simulink library "SimplusGT_2020a"  (R2020a)
settings: Solver=ode45  StartTime=0.0  StopTime=10.0  RelTol=1e-3
undefined symbols (not defined in the file): ang_r, Cf, DiscIntNeverNeededParam, initial, Lc, Lf, m, OtherInputs, P_dc, Sbase, t0, Tm_pu, Ts, V, Vbase, w_droop, w_i, w_pll, w_tau, w_v, Wbase, wc, wfil, x0, Ybase, Zbase
libraries: powerlib x217, $bdroot x1, SimplexPS_2015a x1
(part 3 of 5)

== system SimplusGT_2020a/P-w droop ==
  note: p-w droop controller
      |
      | Author(s): Yitong Li
      |
      | Notes:
      |
      | The power reference should be in source convention.
  pq : Inport
  Constant : Constant  Value=w0
  Constant2 : Constant  Value=theta0
  Constant4 : Constant  Value=2*pi
  Constant6 : Constant  Value=p0
  Demux : Demux  Outputs=2
  Discrete-Time Integrator : DiscreteIntegrator  SampleTime=Ts  ICPrevOutput=DiscIntNeverNeededParam  ICPrevScaledInput=DiscIntNeverNeededParam
  Filter p : DiscreteTransferFcn  Numerator=w_tau*Ts  Denominator=[1 ((w_tau*Ts)-1)]  SampleTime=Ts
  Gain : Gain  Gain=1/Sbase
  Gain2 : Gain  Gain=m
  Gain3 : Gain  Gain=Wbase
  Math Function1 : Math  Operator=mod  SignedPower=on  SaturateOnIntegerOverflow=on
  Sum : Sum
  Sum1 : Sum
  Sum2 : Sum  Inputs=+-
  w : Outport
  theta : Outport  Port=2
  wires:
  Gain3/1 -> Discrete-Time Integrator/1, w/1, [w]
  Sum/1 -> Gain3/1
  Sum2/1 -> Gain2/1
  Constant6/1 -> Sum2/1
  pq/1 -> Demux/1
  Constant4/1 -> Math Function1/2
  Constant/1 -> Sum/2
  Filter p/1 -> Sum2/2
  Discrete-Time Integrator/1 -> Sum1/1
  Gain2/1 -> Sum/1
  Math Function1/1 -> theta/1, [theta]
  Constant2/1 -> [theta0], Sum1/2
  Sum1/1 -> Math Function1/1
  Demux/1 -> Gain/1  "p"
  Gain/1 -> Filter p/1

== system SimplusGT_2020a/PLL (vDQ -> vq) ==
  note: Gpll
  note: Measurement
  note: Phase lock loop (PLL)
      |
      | Author(s): Yitong Li
      |
      | Notes:
      |
      | vq is fed into the PI controller of the PLL.
      |
      | This PLL assumes the input voltage is in DQ frame, which is the common electrical frame. It is not a practical PLL which uses vabc as the input. But this PLL is useful in research.
  vDQ : Inport
  wDQ : Inport  Port=2
  Constant1 : Constant
  Constant2 : Constant  Value=theta0
  Constant3 : Constant
  Constant4 : Constant  Value=2*pi
  Constant6 : Constant  Value=0
  Demux1 : Demux  Outputs=2
  Discrete PI1 : Subsystem  AncestorBlock=SimplusGT/Discrete PI  mask{Kp=w_pll, Ki=w_pll*w_pll/4, xmax=inf, xmin=-inf, Ts=Ts}
      mask prompts: Kp "Proportional Gain"; Ki "Integral Gain"; xmax "Upper Limit"; xmin "Lower Limit"; Ts "Sampling Time"
  Discrete-Time Integrator : DiscreteIntegrator  SampleTime=Ts  ICPrevOutput=DiscIntNeverNeededParam  ICPrevScaledInput=DiscIntNeverNeededParam
  Filter p : DiscreteTransferFcn  Numerator=w_tau*Ts  Denominator=[1 ((w_tau*Ts)-1)]  SampleTime=Ts
  Gain1 : Gain  Gain=Wbase
  Gain2 : Gain  Gain=1/Vbase
  Gain4 : Gain  Gain=1/Wbase
  Gain5 : Gain  Gain=1/pi
  Math Function1 : Math  Operator=mod  SignedPower=on  SaturateOnIntegerOverflow=on
  Mux : Mux  Inputs=2
  Scope : Scope  NumInputPorts=4
  Sum : Sum
  Sum1 : Sum
  Sum2 : Sum  Inputs=+-
  "x1y1 -> x2y2" : Subsystem  AncestorBlock=SimplusGT/x1y1 -> x2y2
  wdq : Outport
  theta : Outport  Port=2
  vdq : Outport  Port=3
  wires:
  [theta0] -> Mux/1  "theta0"
  Constant2/1 -> [theta0], Sum1/2
  Math Function1/1 -> "x1y1 -> x2y2"/2(theta), theta/1, [theta]
  Sum1/1 -> Math Function1/1
  Demux1/2 -> [vq], Gain2/1
  vDQ/1 -> "x1y1 -> x2y2"/1(x1y1)
  Discrete-Time Integrator/1 -> Sum1/1
  Gain2/1 -> Filter p/1
  [vd] -> Scope/1  "vd"
  Mux/1 -> Gain5/1
  Discrete PI1/1(Out) -> Sum/1
  "x1y1 -> x2y2"/1(x2y2) -> vdq/1, Demux1/1
  [w] -> Gain4/1  "w"
  Constant4/1 -> Math Function1/2
  [theta] -> Mux/2  "theta"
  Demux1/1 -> [vd]
  Gain5/1 -> Scope/4
  Constant1/1 -> Discrete PI1/1(enable)
  Gain4/1 -> Scope/3
  Gain1/1 -> Sum/2
  Constant3/1 -> Gain1/1
  [vq] -> Scope/2  "vq"
  Filter p/1 -> Discrete PI1/2(reference)
  Constant6/1 -> Discrete PI1/4(actual), Discrete PI1/3(initial)
  Sum/1 -> Sum2/1
  Sum2/1 -> [w], wdq/1, Discrete-Time Integrator/1
  wDQ/1 -> Sum2/2

== system SimplusGT_2020a/PLL (vabc -> theta) ==
  note: Measurement
  note: Gpll
  note: Phase lock loop (PLL)
      |
      | Author(s): Yitong Li
      |
      | Notes:
      |
      | theta of voltage is fed into the PI controller of the PLL.
  vabc : Inport
  Constant1 : Constant
  Constant2 : Constant  Value=2*pi
  Constant3 : Constant  Value=0
  Constant4 : Constant
  Constant5 : Constant  Value=theta0
  Demux : Demux  Outputs=2
  Discrete PI : Subsystem  AncestorBlock=SimplusGT/Discrete PI  mask{Kp=w_pll, Ki=w_pll*w_pll/4, xmax=inf, xmin=-inf, Ts=Ts}
      mask prompts: Kp "Proportional Gain"; Ki "Integral Gain"; xmax "Upper Limit"; xmin "Lower Limit"; Ts "Sampling Time"
  Discrete-Time Integrator : DiscreteIntegrator  SampleTime=Ts  ICPrevOutput=DiscIntNeverNeededParam  ICPrevScaledInput=DiscIntNeverNeededParam
  Filter p : DiscreteTransferFcn  Numerator=w_tau*Ts  Denominator=[1 ((w_tau*Ts)-1)]  SampleTime=Ts
  Gain1 : Gain  Gain=Wbase
  Gain4 : Gain  Gain=1/Wbase
  Gain5 : Gain  Gain=1/pi
  Math Function1 : Math  Operator=mod  SignedPower=on  SaturateOnIntegerOverflow=on
  Mux : Mux  Inputs=2
  Scope : Scope  NumInputPorts=4
  Selector : Selector  InputPortWidth=2  IndexOptions=Index vector (dialog)  Indices=[2 1]  OutputSizes=1
  Sum : Sum
  Sum1 : Sum
  Trigonometric Function : Trigonometry  Operator=atan2
  "abc -> dq (Power-Invariant)" : Subsystem  AncestorBlock=|
      | SimplusGT/abc -> dq
      | (Power-Invariant)
  w : Outport
  theta : Outport  Port=2
  vdq : Outport  Port=3
  wires:
  Constant2/1 -> Math Function1/2
  Constant1/1 -> Discrete PI/1(enable)
  Constant3/1 -> Discrete PI/3(initial), Discrete PI/4(actual)
  Trigonometric Function/1 -> Filter p/1
  Demux/1 -> [vq], Trigonometric Function/1
  Demux/2 -> [vd], Trigonometric Function/2
  Selector/1 -> Demux/1
  Math Function1/1 -> "abc -> dq (Power-Invariant)"/2(theta), [theta], theta/1
  "abc -> dq (Power-Invariant)"/1(dq) -> vdq/1, Selector/1
  vabc/1 -> "abc -> dq (Power-Invariant)"/1(abc)
  Discrete PI/1(Out) -> Sum/1
  Constant4/1 -> Gain1/1
  Sum/1 -> [w], w/1, Discrete-Time Integrator/1
  Filter p/1 -> Discrete PI/2(reference)
  [vq] -> Scope/2  "vq"
  Mux/1 -> Gain5/1
  [vd] -> Scope/1  "vd"
  [theta] -> Mux/2  "theta"
  Gain5/1 -> Scope/4
  Gain4/1 -> Scope/3
  [w] -> Gain4/1  "w"
  [theta0] -> Mux/1  "theta0"
  Gain1/1 -> Sum/2
  Discrete-Time Integrator/1 -> Sum1/1
  Sum1/1 -> Math Function1/1
  Constant5/1 -> [theta0], Sum1/2

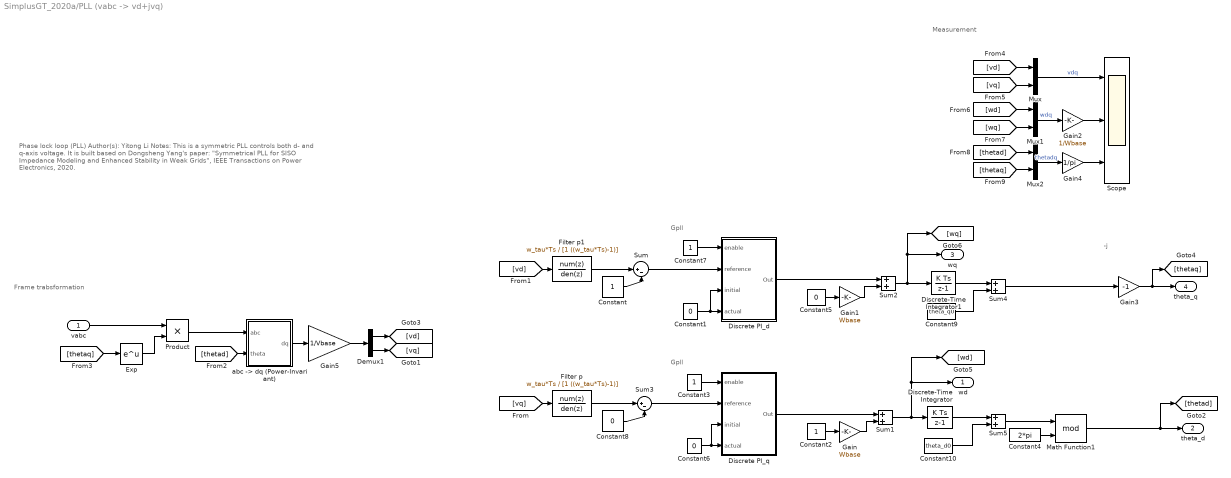
== system SimplusGT_2020a/PLL (vabc -> vd+jvq) ==
  note: Measurement
  note: Frame trabsformation
  note: -j
  note: Gpll
  note: Gpll
  note: Phase lock loop (PLL)
      |
      | Author(s): Yitong Li
      |
      | Notes:
      |
      | This is a symmetric PLL controls both d- and q-axis voltage.
      |
      | It is built based on Dongsheng Yang's paper: "Symmetrical PLL for SISO Impedance Modeling and Enhanced Stability in Weak Grids", IEEE Transactions on Power Electronics, 2020.
  vabc : Inport
  Constant{,2..3,7} (4 alike) : Constant
  Constant{1,5..6,8} (4 alike) : Constant  Value=0
  Constant10 : Constant  Value=theta_d0
  Constant4 : Constant  Value=2*pi
  Constant9 : Constant  Value=theta_q0
  Demux1 : Demux  Outputs=2
  Discrete PI_d : Subsystem  AncestorBlock=SimplusGT/Discrete PI  mask{Kp=w_pll, Ki=w_pll*w_pll/4, xmax=inf, xmin=-inf, Ts=Ts}
      mask prompts: Kp "Proportional Gain"; Ki "Integral Gain"; xmax "Upper Limit"; xmin "Lower Limit"; Ts "Sampling Time"
  Discrete PI_q : Subsystem  AncestorBlock=SimplusGT/Discrete PI  mask{Kp=w_pll, Ki=w_pll*w_pll/4, xmax=inf, xmin=-inf, Ts=Ts}
      mask prompts: Kp "Proportional Gain"; Ki "Integral Gain"; xmax "Upper Limit"; xmin "Lower Limit"; Ts "Sampling Time"
  Discrete-Time Integrator : DiscreteIntegrator  SampleTime=Ts  ICPrevOutput=DiscIntNeverNeededParam  ICPrevScaledInput=DiscIntNeverNeededParam
  Discrete-Time Integrator1 : DiscreteIntegrator  SampleTime=Ts  ICPrevOutput=DiscIntNeverNeededParam  ICPrevScaledInput=DiscIntNeverNeededParam
  Exp : Math  SignedPower=on  SaturateOnIntegerOverflow=on
  Filter p : DiscreteTransferFcn  Numerator=w_tau*Ts  Denominator=[1 ((w_tau*Ts)-1)]  SampleTime=Ts
  Filter p1 : DiscreteTransferFcn  Numerator=w_tau*Ts  Denominator=[1 ((w_tau*Ts)-1)]  SampleTime=Ts
  Gain : Gain  Gain=Wbase
  Gain1 : Gain  Gain=Wbase
  Gain2 : Gain  Gain=1/Wbase
  Gain3 : Gain  Gain=-1
  Gain4 : Gain  Gain=1/pi
  Gain5 : Gain  Gain=1/Vbase
  Math Function1 : Math  Operator=mod  SignedPower=on  SaturateOnIntegerOverflow=on
  Mux : Mux  Inputs=2
  Mux1 : Mux  Inputs=2
  Mux2 : Mux  Inputs=2
  Product : Product
  Scope : Scope  NumInputPorts=3
  Sum : Sum  Inputs=|+-
  Sum{1..2,4..5} (4 alike) : Sum
  Sum3 : Sum  Inputs=|+-
  "abc -> dq (Power-Invariant)" : Subsystem  AncestorBlock=|
      | SimplusGT/abc -> dq
      | (Power-Invariant)
  wd : Outport
  theta_d : Outport  Port=2
  wq : Outport  Port=3
  theta_q : Outport  Port=4
  wires:
  Constant4/1 -> Math Function1/2
  Constant6/1 -> Discrete PI_q/3(initial), Discrete PI_q/4(actual)
  Demux1/2 -> [vq]
  Constant3/1 -> Discrete PI_q/1(enable)
  Math Function1/1 -> theta_d/1, [thetad]
  "abc -> dq (Power-Invariant)"/1(dq) -> Gain5/1
  Gain5/1 -> Demux1/1
  Demux1/1 -> [vd]
  Constant/1 -> Sum/2
  Sum/1 -> Discrete PI_d/2(reference)
  Constant7/1 -> Discrete PI_d/1(enable)
  Constant1/1 -> Discrete PI_d/4(actual), Discrete PI_d/3(initial)
  [thetad] -> "abc -> dq (Power-Invariant)"/2(theta)
  vabc/1 -> Product/1
  Product/1 -> "abc -> dq (Power-Invariant)"/1(abc)
  Exp/1 -> Product/2
  Gain3/1 -> theta_q/1, [thetaq]
  [vq] -> Filter p/1
  [vd] -> Filter p1/1
  Filter p1/1 -> Sum/1
  [thetaq] -> Exp/1
  Sum1/1 -> [wd], wd/1, Discrete-Time Integrator/1
  Discrete PI_q/1(Out) -> Sum1/1
  Sum2/1 -> Discrete-Time Integrator1/1, wq/1, [wq]
  Discrete PI_d/1(Out) -> Sum2/1
  Constant2/1 -> Gain/1
  Constant5/1 -> Gain1/1
  Filter p/1 -> Sum3/1
  Constant8/1 -> Sum3/2
  Sum3/1 -> Discrete PI_q/2(reference)
  Discrete-Time Integrator1/1 -> Sum4/1
  Sum4/1 -> Gain3/1
  Constant9/1 -> Sum4/2
  Gain/1 -> Sum1/2
  Gain1/1 -> Sum2/2
  Discrete-Time Integrator/1 -> Sum5/1
  Sum5/1 -> Math Function1/1
  Constant10/1 -> Sum5/2
  [vd] -> Mux/1
  [vq] -> Mux/2
  [wd] -> Mux1/1
  [wq] -> Mux1/2
  [thetad] -> Mux2/1
  [thetaq] -> Mux2/2
  Mux/1 -> Scope/1  "vdq"
  Mux1/1 -> Gain2/1  "wdq"
  Mux2/1 -> Gain4/1  "thetadq"
  Gain2/1 -> Scope/2
  Gain4/1 -> Scope/3

== system SimplusGT_2020a/PLL (vabc -> vq) ==
  note: Measurement
  note: Gpll
  note: Phase lock loop (PLL)
      |
      | Author(s): Yitong Li
      |
      | Notes:
      |
      | vq is fed into the PI controller of the PLL.
  vabc : Inport
  Constant1 : Constant
  Constant2 : Constant  Value=theta0
  Constant3 : Constant
  Constant4 : Constant  Value=2*pi
  Constant6 : Constant  Value=0
  Demux1 : Demux  Outputs=2
  Discrete PI : Subsystem  AncestorBlock=SimplusGT/Discrete PI  mask{Kp=w_pll, Ki=w_pll*w_pll/4, xmax=inf, xmin=-inf, Ts=Ts}
      mask prompts: Kp "Proportional Gain"; Ki "Integral Gain"; xmax "Upper Limit"; xmin "Lower Limit"; Ts "Sampling Time"
  Discrete-Time Integrator : DiscreteIntegrator  SampleTime=Ts  ICPrevOutput=DiscIntNeverNeededParam  ICPrevScaledInput=DiscIntNeverNeededParam
  Filter p : DiscreteTransferFcn  Numerator=w_tau*Ts  Denominator=[1 ((w_tau*Ts)-1)]  SampleTime=Ts
  Gain1 : Gain  Gain=Wbase
  Gain2 : Gain  Gain=1/Vbase
  Gain4 : Gain  Gain=1/Wbase
  Gain5 : Gain  Gain=1/pi
  Math Function1 : Math  Operator=mod  SignedPower=on  SaturateOnIntegerOverflow=on
  Mux : Mux  Inputs=2
  Scope : Scope  NumInputPorts=4
  Sum : Sum
  Sum1 : Sum
  "abc -> dq (Power-Invariant)" : Subsystem  AncestorBlock=|
      | SimplusGT/abc -> dq
      | (Power-Invariant)
  w : Outport
  theta : Outport  Port=2
  vdq : Outport  Port=3
  wires:
  vabc/1 -> "abc -> dq (Power-Invariant)"/1(abc)
  "abc -> dq (Power-Invariant)"/1(dq) -> vdq/1, Demux1/1
  Constant4/1 -> Math Function1/2
  Gain2/1 -> Filter p/1
  Demux1/2 -> [vq], Gain2/1
  Constant6/1 -> Discrete PI/4(actual), Discrete PI/3(initial)
  Constant1/1 -> Discrete PI/1(enable)
  Discrete PI/1(Out) -> Sum/1
  Sum/1 -> [w], w/1, Discrete-Time Integrator/1
  Gain1/1 -> Sum/2
  Discrete-Time Integrator/1 -> Sum1/1
  Sum1/1 -> Math Function1/1
  Constant2/1 -> [theta0], Sum1/2
  Filter p/1 -> Discrete PI/2(reference)
  [vq] -> Scope/2  "vq"
  Mux/1 -> Gain5/1
  Gain4/1 -> Scope/3
  [w] -> Gain4/1  "w"
  [theta0] -> Mux/1  "theta0"
  [vd] -> Scope/1  "vd"
  Gain5/1 -> Scope/4
  [theta] -> Mux/2  "theta"
  Demux1/1 -> [vd]
  Constant3/1 -> Gain1/1
  Math Function1/1 -> "abc -> dq (Power-Invariant)"/2(theta), [theta], theta/1

== system SimplusGT_2020a/PQ Calculation (dq-Frame) ==
  note: Power calculation.
      |
      | Author(s): Yitong Li
      |
      | Notes:
      |
      | The calculation is done in dq frame.
  vdq : Inport
  idq : Inport  Port=2
  Mux : Mux  Inputs=2
  Mux1 : Mux  Inputs=2
  P = vd*id+vq*iq : Fcn  Expr=u[1]*u[3]+u[2]*u[4]
  Q = -vd*iq+vq*id : Fcn  Expr=-u[1]*u[4]+u[2]*u[3]
  pq : Outport
  wires:
  Q = -vd*iq+vq*id/1 -> Mux/2
  Mux1/1 -> Q = -vd*iq+vq*id/1, P = vd*id+vq*iq/1
  idq/1 -> Mux1/2
  vdq/1 -> Mux1/1
  P = vd*id+vq*iq/1 -> Mux/1
  Mux/1 -> pq/1

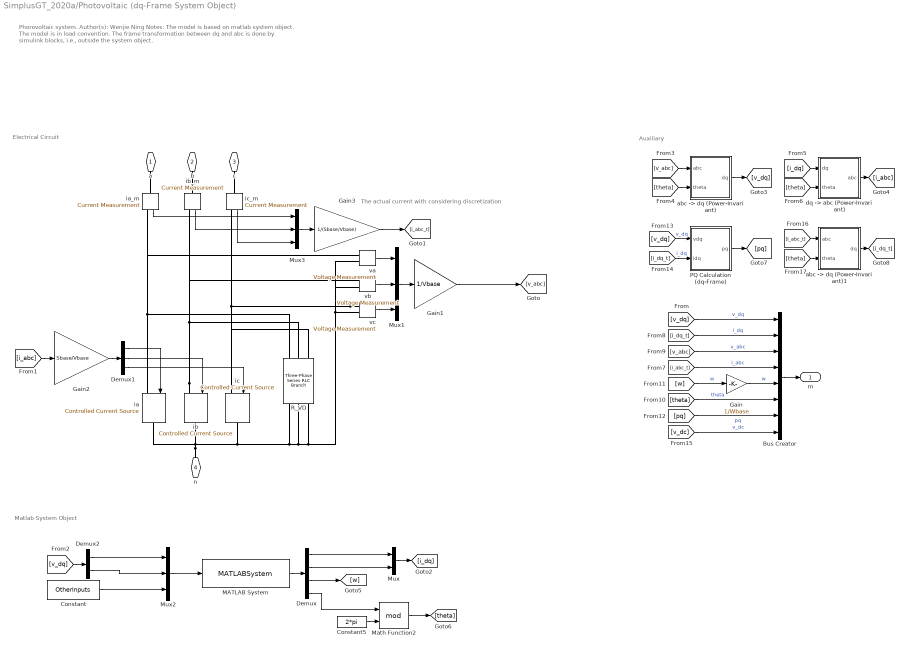
== system SimplusGT_2020a/Photovoltaic (dq-Frame System Object) ==
  note: The actual current with considering discretization
  note: Phorovoltaic system.
      |
      | Author(s): Wenjie Ning
      |
      | Notes:
      |
      | The model is based on matlab system object.
      |
      | The model is in load convention.
      |
      | The frame transformation between dq and abc is done by simulink blocks, i.e., outside the system object.
  note: Electrical Circuit
  note: Auxiliary
  note: Matlab System Object
  Bus Creator : BusCreator  Inputs=8
  Constant : Constant  Value=OtherInputs
  Constant5 : Constant  Value=2*pi
  Demux : Demux
  Demux1 : Demux  Outputs=3
  Demux2 : Demux  Outputs=2
  Gain : Gain  Gain=1/Wbase
  Gain1 : Gain  Gain=1/Vbase
  Gain2 : Gain  Gain=Sbase/Vbase
  Gain3 : Gain  Gain=1/(Sbase/Vbase)
  MATLAB System : MATLABSystem  System=SimplusGT.Class.Photovoltaic  Ts=Ts  Para=ApparatusPara  ApparatusType=ApparatusType  PowerFlow=PowerFlow  x0=x0  DiscreMethod=DiscreMethod  LinearizationTimes=LinearizationTimes  DirectFeedthrough=DirectFeedthrough  VirtualResistor=DiscreDampingFlag  EquiInitial=true  ElecPortIOs=[ 1, 2 ]  SimulateUsing=Code generation
      mask Type: SimplusGT.Class.Photovoltaic
      mask Display:
      | disp('Photovoltaic');
      | port_label('input',1,'u');
      | port_label('output',1,'y');
  Math Function2 : Math  Operator=mod  SignedPower=on  SaturateOnIntegerOverflow=on
  Mux : Mux  Inputs=2
  Mux1 : Mux  Inputs=3
  Mux2 : Mux  Inputs=3
  Mux3 : Mux  Inputs=3
  PQ Calculation (dq-Frame) : Subsystem  AncestorBlock=|
      | SimplusGT/PQ Calculation
      | (dq-Frame)
  R_VD : powerlib/Elements/Three-Phase Series RLC Branch  LConnTagsString=A|B|C  RConnTagsString=A|B|C  BranchType=R  Resistance=DiscreDampingValue*Vbase^2/Sbase  Inductance=1e-3  Capacitance=1e-6  Measurements=None
  "abc -> dq (Power-Invariant)" : Subsystem  AncestorBlock=|
      | SimplusGT/abc -> dq
      | (Power-Invariant)
  "abc -> dq (Power-Invariant)1" : Subsystem  AncestorBlock=|
      | SimplusGT/abc -> dq
      | (Power-Invariant)
  "dq -> abc (Power-Invariant)" : Subsystem  AncestorBlock=|
      | SimplusGT/dq -> abc
      | (Power-Invariant)
  ia : powerlib/Electrical Sources/Controlled Current Source  Initialize=on  Source_Type=AC  Amplitude=0  Phase=0  Frequency=0  Measurements=None
  ia_m : powerlib/Measurements/Current Measurement  PhasorSimulation=off  OutputType=Complex  PSBequivalent=0
  ib : powerlib/Electrical Sources/Controlled Current Source  Initialize=on  Source_Type=AC  Amplitude=0  Phase=0  Frequency=0  Measurements=None
  ib_m : powerlib/Measurements/Current Measurement  PhasorSimulation=off  OutputType=Complex  PSBequivalent=0
  ic : powerlib/Electrical Sources/Controlled Current Source  Initialize=on  Source_Type=AC  Amplitude=0  Phase=0  Frequency=0  Measurements=None
  ic_m : powerlib/Measurements/Current Measurement  PhasorSimulation=off  OutputType=Complex  PSBequivalent=0
  va : powerlib/Measurements/Voltage Measurement  PhasorSimulation=off  OutputType=Complex  PSBequivalent=0
  vb : powerlib/Measurements/Voltage Measurement  PhasorSimulation=off  OutputType=Complex  PSBequivalent=0
  vc : powerlib/Measurements/Voltage Measurement  PhasorSimulation=off  OutputType=Complex  PSBequivalent=0
  a : PMIOPort  Side=Left
  b : PMIOPort  Port=2  Side=Left
  c : PMIOPort  Port=3  Side=Left
  n : PMIOPort  Port=4  Side=Left
  m : Outport
  wires:
  "abc -> dq (Power-Invariant)1"/1(dq) -> [i_dq_t]
  [theta] -> "abc -> dq (Power-Invariant)1"/2(theta)
  [i_abc_t] -> "abc -> dq (Power-Invariant)1"/1(abc)
  Mux3/1 -> Gain3/1
  Gain3/1 -> [i_abc_t]
  ib_m/1 -> Mux3/2
  ia_m/1 -> Mux3/1
  ic_m/1 -> Mux3/3
  Constant/1 -> Mux2/3
  Demux/4 -> Math Function2/1
  [v_dc] -> Bus Creator/8  "v_dc"
  Gain1/1 -> [v_abc]
  Gain2/1 -> Demux1/1
  PQ Calculation (dq-Frame)/1(pq) -> [pq]
  [i_dq_t] -> PQ Calculation (dq-Frame)/2(idq)  "i_dq"
  [v_dq] -> PQ Calculation (dq-Frame)/1(vdq)  "v_dq"
  [pq] -> Bus Creator/7  "pq"
  [i_abc] -> Gain2/1
  Gain/1 -> Bus Creator/5  "w"
  [w] -> Gain/1  "w"
  Bus Creator/1 -> m/1
  Math Function2/1 -> [theta]
  Constant5/1 -> Math Function2/2
  Demux1/3 -> ic/1
  vc/1 -> Mux1/3
  MATLAB System/1 -> Demux/1
  Mux2/1 -> MATLAB System/1
  "dq -> abc (Power-Invariant)"/1(abc) -> [i_abc]
  [theta] -> "dq -> abc (Power-Invariant)"/2(theta)
  [i_dq] -> "dq -> abc (Power-Invariant)"/1(dq)
  "abc -> dq (Power-Invariant)"/1(dq) -> [v_dq]
  [theta] -> "abc -> dq (Power-Invariant)"/2(theta)
  [v_abc] -> "abc -> dq (Power-Invariant)"/1(abc)
  [theta] -> Bus Creator/6  "theta"
  [i_abc_t] -> Bus Creator/4  "i_abc"
  [v_abc] -> Bus Creator/3  "v_abc"
  [i_dq_t] -> Bus Creator/2  "i_dq"
  [v_dq] -> Bus Creator/1  "v_dq"
  Demux2/2 -> Mux2/2
  Demux2/1 -> Mux2/1
  [v_dq] -> Demux2/1
  Mux1/1 -> Gain1/1
  vb/1 -> Mux1/2
  va/1 -> Mux1/1
  Demux1/2 -> ib/1
  Demux1/1 -> ia/1
  Demux/3 -> [w]
  Mux/1 -> [i_dq]
  Demux/1 -> Mux/1
  Demux/2 -> Mux/2
  connections:
  ic_m/LConn1 -- c/RConn1
  ib_m/LConn1 -- b/RConn1
  ia_m/LConn1 -- a/RConn1
  vc/LConn1 -- ic_m/RConn1 -- ic/LConn1 -- R_VD/LConn3
  ib/LConn1 -- vb/LConn1 -- ib_m/RConn1 -- R_VD/LConn2
  ia/LConn1 -- ia_m/RConn1 -- va/LConn1 -- R_VD/LConn1
  n/RConn1 -- ib/RConn1 -- ia/RConn1 -- ic/RConn1 -- R_VD/RConn1 -- R_VD/RConn2 -- R_VD/RConn3 -- vc/LConn2 -- va/LConn2 -- vb/LConn2

== system SimplusGT_2020a/ReIm2Complex ==
  note: Transformation from real/imaginary to complex vectors
      |
      | Author(s): Yitong Li
      |
      | Notes:
      |
      | A example is from dq frame to dq+- frame.
  Re Im : Inport
  -> backward : Fcn  Expr=u[1] - u[2]*1i
  -> forward : Fcn  Expr=u[1] + u[2]*1i
  Mux : Mux  Inputs=2
  +- : Outport
  wires:
  Re Im/1 -> -> backward/1, -> forward/1
  Mux/1 -> +-/1
  -> forward/1 -> Mux/1
  -> backward/1 -> Mux/2

== system SimplusGT_2020a/Root Mean Squre ==
  note: Root mean squre
      |
      | Author(s): Yitong Li
  x : Inport
  y : Inport  Port=2
  Math Function1 : Math  Operator=square  SignedPower=on  SaturateOnIntegerOverflow=on
  Math Function2 : Math  Operator=square  SignedPower=on  SaturateOnIntegerOverflow=on
  Sqrt : Sqrt  SaturateOnIntegerOverflow=on
  Sum : Sum
  RMS : Outport
  wires:
  Sum/1 -> Sqrt/1
  x/1 -> Math Function1/1
  Sqrt/1 -> RMS/1
  Math Function1/1 -> Sum/1
  y/1 -> Math Function2/1
  Math Function2/1 -> Sum/2

== system SimplusGT_2020a/Single Pulse ==
  note: Pulse generator
      |
      | Author(s): Yitong Li
  Gain : Gain  Gain=Am
  Product : Product
  Step : Step  Time=t0  SampleTime=0
  Step1 : Step  Time=t0+dt  Before=1  After=0  SampleTime=0
  Out : Outport
  wires:
  Step1/1 -> Product/2
  Step/1 -> Product/1
  Product/1 -> Gain/1
  Gain/1 -> Out/1

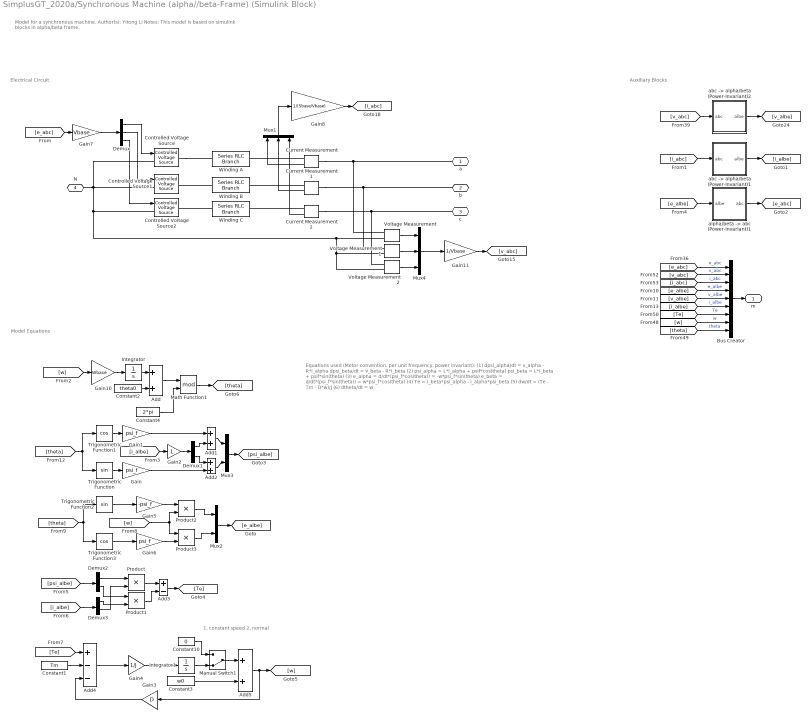
== system SimplusGT_2020a/Synchronous Machine (alpha//beta-Frame) (Simulink Block) ==
  note: 1. constant speed
      | 2. normal
  note: Auxiliary Blocks
  note: Model Equations
  note: Electrical Circuit
  note: Equations used
      | (Motor convention, per unit frequency, power invariant):
      |
      | (1) dpsi_alpha/dt = v_alpha - R*i_alpha
      | dpsi_beta/dt = v_beta - R*i_beta
      |
      | (2) psi_alpha = L*i_alpha + psif*cos(theta)
      | psi_beta = L*i_beta + psif*sin(theta)
      |
      | (3) e_alpha = d/dt*(psi_f*cos(theta)) = -w*psi_f*sin(theta)
      | e_beta = d/dt*(psi_f*sin(theta)) = w*psi_f*cos(theta)
      |
      | (4) Te = i_beta*psi_alpha - i_alpha*psi_beta
      | (5) dw/dt = (Te - Tm - D*w)/J
      | (6) dtheta/dt = w
  note: Model for a synchronous machine.
      |
      | Author(s): Yitong Li
      |
      | Notes:
      |
      | This model is based on simulink blocks in alpha/beta frame.
  Add{,1..2,5} (4 alike) : Sum
  Add3 : Sum  Inputs=+-
  Add4 : Sum  Inputs=+--
  Bus Creator : BusCreator  Inputs=9
  Constant1 : Constant  Value=Tm
  Constant10 : Constant  Value=0
  Constant2 : Constant  Value=theta0
  Constant3 : Constant  Value=w0
  Constant4 : Constant  Value=2*pi
  Controlled Voltage Source : powerlib/Electrical Sources/Controlled Voltage Source  Initialize=on  Source_Type=AC  Amplitude=0  Phase=0  Frequency=0  Measurements=None
  Controlled Voltage Source1 : powerlib/Electrical Sources/Controlled Voltage Source  Initialize=on  Source_Type=AC  Amplitude=0  Phase=0  Frequency=0  Measurements=None
  Controlled Voltage Source2 : powerlib/Electrical Sources/Controlled Voltage Source  Initialize=on  Source_Type=AC  Amplitude=0  Phase=0  Frequency=0  Measurements=None
  Current Measurement : powerlib/Measurements/Current Measurement  PhasorSimulation=off  OutputType=Complex  PSBequivalent=0
  Current Measurement1 : powerlib/Measurements/Current Measurement  PhasorSimulation=off  OutputType=Complex  PSBequivalent=0
  Current Measurement2 : powerlib/Measurements/Current Measurement  PhasorSimulation=off  OutputType=Complex  PSBequivalent=0
  Demux : Demux  Outputs=3
  Demux1 : Demux  Outputs=2
  Demux2 : Demux  Outputs=2
  Demux3 : Demux  Outputs=2
  Gain : Gain  Gain=psi_f
  Gain1 : Gain  Gain=psi_f
  Gain10 : Gain  Gain=Wbase
  Gain11 : Gain  Gain=1/Vbase
  Gain2 : Gain  Gain=L
  Gain3 : Gain  Gain=D
  Gain4 : Gain  Gain=1/J
  Gain5 : Gain  Gain=-psi_f
  Gain6 : Gain  Gain=psi_f
  Gain7 : Gain  Gain=Vbase
  Gain8 : Gain  Gain=1/(Sbase/Vbase)
  Integrator : Integrator
  Integrator1 : Integrator
  Manual Switch1 : ManualSwitch  CurrentSetting=0
  Math Function1 : Math  Operator=mod  SignedPower=on  SaturateOnIntegerOverflow=on
  Mux1 : Mux  Inputs=3
  Mux2 : Mux  Inputs=2
  Mux3 : Mux  Inputs=2
  Mux4 : Mux  Inputs=3
  Product{,1..3} (4 alike) : Product
  Trigonometric Function : Trigonometry
  Trigonometric Function1 : Trigonometry  Operator=cos
  Trigonometric Function2 : Trigonometry
  Trigonometric Function3 : Trigonometry  Operator=cos
  Voltage Measurement : powerlib/Measurements/Voltage Measurement  PhasorSimulation=off  OutputType=Complex  PSBequivalent=0
  Voltage Measurement1 : powerlib/Measurements/Voltage Measurement  PhasorSimulation=off  OutputType=Complex  PSBequivalent=0
  Voltage Measurement2 : powerlib/Measurements/Voltage Measurement  PhasorSimulation=off  OutputType=Complex  PSBequivalent=0
  Winding A : powerlib/Elements/Series RLC Branch  LConnTagsString=__new0  RConnTagsString=__new0  BranchType=RL  Resistance=R*(Vbase^2)/Sbase  Inductance=L*(Vbase^2)/Sbase/Wbase  SetiL0=off  InitialCurrent=ia0  Capacitance=1e-6  Setx0=off  InitialVoltage=0  Measurements=None
  Winding B : powerlib/Elements/Series RLC Branch  LConnTagsString=__new0  RConnTagsString=__new0  BranchType=RL  Resistance=R*(Vbase^2)/Sbase  Inductance=L*(Vbase^2)/Sbase/Wbase  SetiL0=off  InitialCurrent=ia0  Capacitance=1e-6  Setx0=off  InitialVoltage=0  Measurements=None
  Winding C : powerlib/Elements/Series RLC Branch  LConnTagsString=__new0  RConnTagsString=__new0  BranchType=RL  Resistance=R*(Vbase^2)/Sbase  Inductance=L*(Vbase^2)/Sbase/Wbase  SetiL0=off  InitialCurrent=ia0  Capacitance=1e-6  Setx0=off  InitialVoltage=0  Measurements=None
  "abc -> alpha/beta (Power-Invariant)1" : Subsystem  AncestorBlock=|
      | SimplusGT/abc -> alpha//beta
      | (Power-Invariant)
  "abc -> alpha/beta (Power-Invariant)2" : Subsystem  AncestorBlock=|
      | SimplusGT/abc -> alpha//beta
      | (Power-Invariant)
  "alpha/beta -> abc (Power-Invariant)1" : Subsystem  AncestorBlock=|
      | SimplusGT/alpha//beta -> abc
      | (Power-Invariant)
  a : PMIOPort  Side=Left
  b : PMIOPort  Port=2  Side=Left
  c : PMIOPort  Port=3  Side=Left
  N : PMIOPort  Port=4  Side=Left
  m : Outport
  wires:
  Current Measurement/1 -> Mux1/1
  Current Measurement1/1 -> Mux1/2
  Current Measurement2/1 -> Mux1/3
  Mux1/1 -> Gain8/1
  [e_abc] -> Gain7/1
  Demux/1 -> Controlled Voltage Source/1
  Demux/2 -> Controlled Voltage Source1/1
  Demux/3 -> Controlled Voltage Source2/1
  [i_abc] -> "abc -> alpha/beta (Power-Invariant)1"/1(abc)
  "abc -> alpha/beta (Power-Invariant)1"/1(albe) -> [i_albe]
  [w] -> Gain10/1
  Integrator/1 -> Add/1
  Constant2/1 -> Add/2
  Trigonometric Function1/1 -> Gain1/1
  Trigonometric Function/1 -> Gain/1
  [i_albe] -> Gain2/1
  Demux1/1 -> Add1/2
  Demux1/2 -> Add2/1
  Gain2/1 -> Demux1/1
  Gain1/1 -> Add1/1
  Gain/1 -> Add2/2
  Product2/1 -> Mux2/1
  Product3/1 -> Mux2/2
  Mux2/1 -> [e_albe]
  [e_albe] -> "alpha/beta -> abc (Power-Invariant)1"/1(albe)
  "alpha/beta -> abc (Power-Invariant)1"/1(abc) -> [e_abc]
  Add1/1 -> Mux3/1
  Add2/1 -> Mux3/2
  Mux3/1 -> [psi_albe]
  [psi_albe] -> Demux2/1
  [i_albe] -> Demux3/1
  Demux2/1 -> Product/1
  Demux3/2 -> Product/2
  Demux3/1 -> Product1/2
  Demux2/2 -> Product1/1
  Product/1 -> Add3/1
  Product1/1 -> Add3/2
  Add3/1 -> [Te]
  [Te] -> Add4/1
  Constant1/1 -> Add4/2
  Add4/1 -> Gain4/1
  Gain3/1 -> Add4/3
  Constant3/1 -> Add5/2
  Add5/1 -> Gain3/1, [w]
  [theta] -> Trigonometric Function3/1, Trigonometric Function2/1
  Trigonometric Function2/1 -> Gain5/1
  Trigonometric Function3/1 -> Gain6/1
  Gain5/1 -> Product2/1
  Gain6/1 -> Product3/2
  Gain8/1 -> [i_abc]
  Gain4/1 -> Integrator1/1
  Gain10/1 -> Integrator/1
  Voltage Measurement/1 -> Mux4/1
  Voltage Measurement1/1 -> Mux4/2
  Voltage Measurement2/1 -> Mux4/3
  Mux4/1 -> Gain11/1
  Gain11/1 -> [v_abc]
  Gain7/1 -> Demux/1
  Add/1 -> Math Function1/1
  Constant4/1 -> Math Function1/2
  Math Function1/1 -> [theta]
  [v_abc] -> "abc -> alpha/beta (Power-Invariant)2"/1(abc)
  "abc -> alpha/beta (Power-Invariant)2"/1(albe) -> [v_albe]
  [w] -> Product3/1, Product2/2
  [theta] -> Trigonometric Function/1, Trigonometric Function1/1
  Integrator1/1 -> Manual Switch1/2
  Manual Switch1/1 -> Add5/1
  Constant10/1 -> Manual Switch1/1
  [e_abc] -> Bus Creator/1  "e_abc"
  [v_abc] -> Bus Creator/2  "v_abc"
  [i_abc] -> Bus Creator/3  "i_abc"
  [e_albe] -> Bus Creator/4  "e_albe"
  [v_albe] -> Bus Creator/5  "v_albe"
  [i_albe] -> Bus Creator/6  "i_albe"
  [Te] -> Bus Creator/7  "Te"
  [w] -> Bus Creator/8  "w"
  [theta] -> Bus Creator/9  "theta"
  Bus Creator/1 -> m/1
  connections:
  Current Measurement/RConn1 -- Winding A/RConn1
  Controlled Voltage Source/RConn1 -- Winding A/LConn1
  Current Measurement2/RConn1 -- Winding C/RConn1
  Current Measurement/LConn1 -- Voltage Measurement/LConn1 -- a/RConn1
  Current Measurement1/LConn1 -- Voltage Measurement1/LConn1 -- b/RConn1
  Current Measurement1/RConn1 -- Winding B/RConn1
  Winding B/LConn1 -- Controlled Voltage Source1/RConn1
  Controlled Voltage Source/LConn1 -- Voltage Measurement2/LConn2 -- Voltage Measurement1/LConn2 -- Voltage Measurement/LConn2 -- Controlled Voltage Source2/LConn1 -- N/RConn1 -- Controlled Voltage Source1/LConn1
  Winding C/LConn1 -- Controlled Voltage Source2/RConn1
  Current Measurement2/LConn1 -- Voltage Measurement2/LConn1 -- c/RConn1

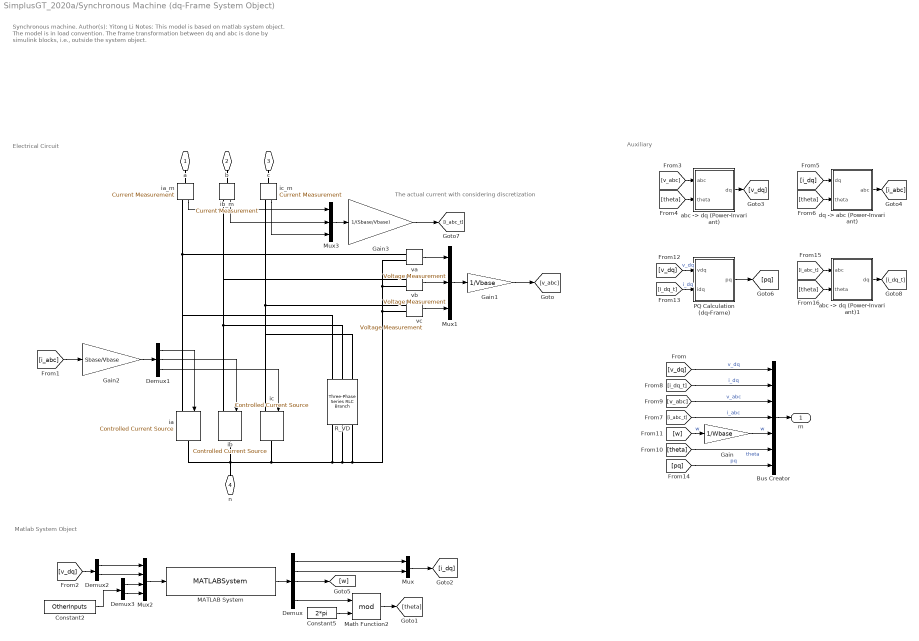
== system SimplusGT_2020a/Synchronous Machine (dq-Frame System Object) ==
  note: The actual current with considering discretization
  note: Synchronous machine.
      |
      | Author(s): Yitong Li
      |
      | Notes:
      |
      | This model is based on matlab system object.
      |
      | The model is in load convention.
      |
      | The frame transformation between dq and abc is done by simulink blocks, i.e., outside the system object.
  note: Matlab System Object
  note: Auxiliary
  note: Electrical Circuit
  Bus Creator : BusCreator  Inputs=7
  Constant2 : Constant  Value=OtherInputs
  Constant5 : Constant  Value=2*pi
  Demux : Demux  Outputs=5
  Demux1 : Demux  Outputs=3
  Demux2 : Demux  Outputs=2
  Demux3 : Demux  Outputs=2
  Gain : Gain  Gain=1/Wbase
  Gain1 : Gain  Gain=1/Vbase
  Gain2 : Gain  Gain=Sbase/Vbase
  Gain3 : Gain  Gain=1/(Sbase/Vbase)
  MATLAB System : MATLABSystem  System=SimplusGT.Class.SynchronousMachine  Ts=Ts  Para=ApparatusPara  ApparatusType=ApparatusType  PowerFlow=PowerFlow  x0=x0  DiscreMethod=DiscreMethod  LinearizationTimes=LinearizationTimes  DirectFeedthrough=DirectFeedthrough  VirtualResistor=DiscreDampingFlag  EquiInitial=true  ElecPortIOs=[ 1, 2 ]  SimulateUsing=Code generation
      mask Type: SimplusGT.Class.SynchronousMachine
      mask Display:
      | disp('SynchronousMachine');
      | port_label('input',1,'u');
      | port_label('output',1,'y');
  Math Function2 : Math  Operator=mod  SignedPower=on  SaturateOnIntegerOverflow=on
  Mux : Mux  Inputs=2
  Mux1 : Mux  Inputs=3
  Mux2 : Mux
  Mux3 : Mux  Inputs=3
  PQ Calculation (dq-Frame) : Subsystem  AncestorBlock=|
      | SimplusGT/PQ Calculation
      | (dq-Frame)
  R_VD : powerlib/Elements/Three-Phase Series RLC Branch  LConnTagsString=A|B|C  RConnTagsString=A|B|C  BranchType=R  Resistance=DiscreDampingValue*Vbase^2/Sbase  Inductance=1e-3  Capacitance=1e-6  Measurements=None
  "abc -> dq (Power-Invariant)" : Subsystem  AncestorBlock=|
      | SimplusGT/abc -> dq
      | (Power-Invariant)
  "abc -> dq (Power-Invariant)1" : Subsystem  AncestorBlock=|
      | SimplusGT/abc -> dq
      | (Power-Invariant)
  "dq -> abc (Power-Invariant)" : Subsystem  AncestorBlock=|
      | SimplusGT/dq -> abc
      | (Power-Invariant)
  ia : powerlib/Electrical Sources/Controlled Current Source  Initialize=on  Source_Type=AC  Amplitude=0  Phase=0  Frequency=0  Measurements=None
  ia_m : powerlib/Measurements/Current Measurement  PhasorSimulation=off  OutputType=Complex  PSBequivalent=0
  ib : powerlib/Electrical Sources/Controlled Current Source  Initialize=on  Source_Type=AC  Amplitude=0  Phase=0  Frequency=0  Measurements=None
  ib_m : powerlib/Measurements/Current Measurement  PhasorSimulation=off  OutputType=Complex  PSBequivalent=0
  ic : powerlib/Electrical Sources/Controlled Current Source  Initialize=on  Source_Type=AC  Amplitude=0  Phase=0  Frequency=0  Measurements=None
  ic_m : powerlib/Measurements/Current Measurement  PhasorSimulation=off  OutputType=Complex  PSBequivalent=0
  va : powerlib/Measurements/Voltage Measurement  PhasorSimulation=off  OutputType=Complex  PSBequivalent=0
  vb : powerlib/Measurements/Voltage Measurement  PhasorSimulation=off  OutputType=Complex  PSBequivalent=0
  vc : powerlib/Measurements/Voltage Measurement  PhasorSimulation=off  OutputType=Complex  PSBequivalent=0
  a : PMIOPort  Side=Left
  b : PMIOPort  Port=2  Side=Left
  c : PMIOPort  Port=3  Side=Left
  n : PMIOPort  Port=4  Side=Left
  m : Outport
  wires:
  Demux/2 -> Mux/2
  Demux/1 -> Mux/1
  Mux/1 -> [i_dq]
  Demux/3 -> [w]
  Demux1/1 -> ia/1
  Demux1/2 -> ib/1
  va/1 -> Mux1/1
  vb/1 -> Mux1/2
  [v_dq] -> Demux2/1
  Demux2/1 -> Mux2/1
  Demux2/2 -> Mux2/2
  [v_abc] -> "abc -> dq (Power-Invariant)"/1(abc)
  [theta] -> "abc -> dq (Power-Invariant)"/2(theta)
  "abc -> dq (Power-Invariant)"/1(dq) -> [v_dq]
  [i_dq] -> "dq -> abc (Power-Invariant)"/1(dq)
  [theta] -> "dq -> abc (Power-Invariant)"/2(theta)
  "dq -> abc (Power-Invariant)"/1(abc) -> [i_abc]
  Mux2/1 -> MATLAB System/1
  MATLAB System/1 -> Demux/1
  vc/1 -> Mux1/3
  Demux1/3 -> ic/1
  Demux/5 -> Math Function2/1
  Constant5/1 -> Math Function2/2
  Math Function2/1 -> [theta]
  [v_dq] -> Bus Creator/1  "v_dq"
  [i_dq_t] -> Bus Creator/2  "i_dq"
  [v_abc] -> Bus Creator/3  "v_abc"
  [i_abc_t] -> Bus Creator/4  "i_abc"
  [w] -> Gain/1  "w"
  [theta] -> Bus Creator/6  "theta"
  Bus Creator/1 -> m/1
  Gain/1 -> Bus Creator/5  "w"
  Mux1/1 -> Gain1/1
  Constant2/1 -> Demux3/1
  Demux3/1 -> Mux2/3
  Demux3/2 -> Mux2/4
  [i_abc] -> Gain2/1
  [v_dq] -> PQ Calculation (dq-Frame)/1(vdq)  "v_dq"
  [i_dq_t] -> PQ Calculation (dq-Frame)/2(idq)  "i_dq"
  PQ Calculation (dq-Frame)/1(pq) -> [pq]
  [pq] -> Bus Creator/7  "pq"
  Gain1/1 -> [v_abc]
  Gain2/1 -> Demux1/1
  ia_m/1 -> Mux3/1
  ib_m/1 -> Mux3/2
  ic_m/1 -> Mux3/3
  Mux3/1 -> Gain3/1
  Gain3/1 -> [i_abc_t]
  [i_abc_t] -> "abc -> dq (Power-Invariant)1"/1(abc)
  [theta] -> "abc -> dq (Power-Invariant)1"/2(theta)
  "abc -> dq (Power-Invariant)1"/1(dq) -> [i_dq_t]
  connections:
  vb/LConn2 -- va/LConn2 -- vc/LConn2 -- R_VD/RConn3 -- R_VD/RConn2 -- R_VD/RConn1 -- ia/RConn1 -- ib/RConn1 -- n/RConn1 -- ic/RConn1
  R_VD/LConn2 -- vb/LConn1 -- ib_m/RConn1 -- ib/LConn1
  R_VD/LConn3 -- ic/LConn1 -- ic_m/RConn1 -- vc/LConn1
  va/LConn1 -- R_VD/LConn1 -- ia/LConn1 -- ia_m/RConn1
  ia_m/LConn1 -- a/RConn1
  ib_m/LConn1 -- b/RConn1
  ic_m/LConn1 -- c/RConn1

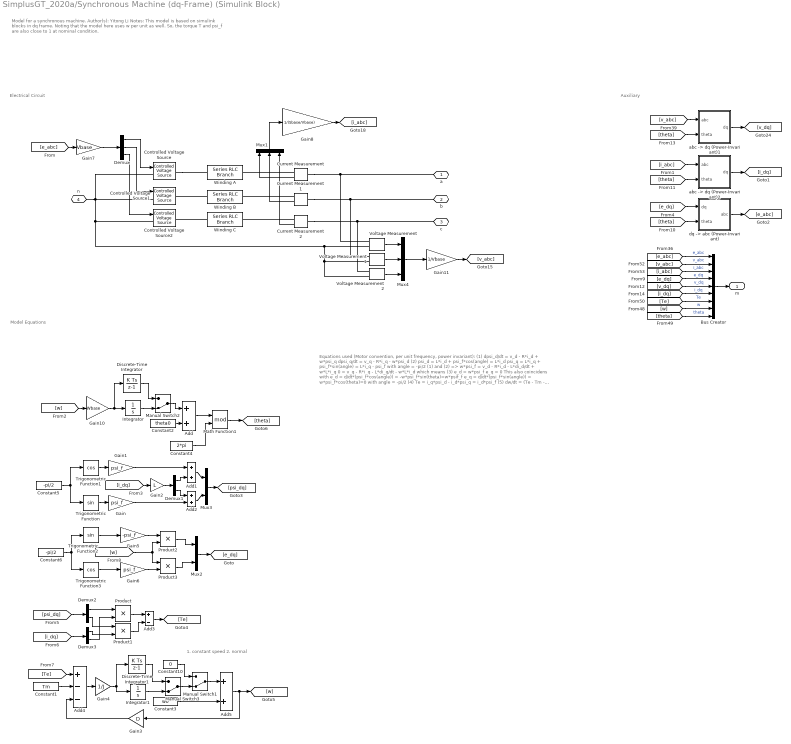
== system SimplusGT_2020a/Synchronous Machine (dq-Frame) (Simulink Block) ==
  note: 1. constant speed
      | 2. normal
  note: Auxiliary
  note: Model Equations
  note: Electrical Circuit
  note: Equations used
      | (Motor convention, per unit frequency, power invariant):
      |
      | (1) dpsi_d/dt = v_d - R*i_d + w*psi_q
      | dpsi_q/dt = v_q - R*i_q - w*psi_d
      |
      | (2) psi_d = L*i_d + psi_f*cos(angle) = L*i_d
      | psi_q = L*i_q + psi_f*sin(angle) = L*i_q - psi_f
      | with angle = -pi/2
      |
      | (1) and (2) =>
      |
      | w*psi_f = v_d - R*i_d - L*di_d/dt + w*L*i_q
      | 0 = v_q - R*i_q - L*di_q/dt - w*L*i_d
      |
      | which means
      |
      | (3) e_d = w*psi_f
      | e_q = 0
      |
      | This also coincidens with
      |
      | e_d = d/dt*(psi_f*cos(angle)) = -w*psi_f*sin(theta)=w*psif_f
      | e_q = d/dt*(psi_f*sin(angle)) = w*psi_f*cos(theta)=0
      | with angle = -pi/2
      |
      | (4) Te = i_q*psi_d - i_d*psi_q = i_d*psi_f
      | (5) dw/dt = (Te - Tm - D*w)/J
      | (6) dtheta/dt = w
  note: Model for a synchronous machine.
      |
      | Author(s): Yitong Li
      |
      | Notes:
      |
      | This model is based on simulink blocks in dq frame.
      |
      | Noting that the model here uses w per unit as well. So, the torque T and psi_f are also close to 1 at nominal condition.
  Add{,1..2,5} (4 alike) : Sum
  Add3 : Sum  Inputs=+-
  Add4 : Sum  Inputs=+--
  Bus Creator : BusCreator  Inputs=9
  Constant1 : Constant  Value=Tm
  Constant10 : Constant  Value=0
  Constant2 : Constant  Value=theta0
  Constant3 : Constant  Value=w0
  Constant4 : Constant  Value=2*pi
  Constant5 : Constant  Value=-pi/2
  Constant6 : Constant  Value=-pi/2
  Controlled Voltage Source : powerlib/Electrical Sources/Controlled Voltage Source  Initialize=on  Source_Type=AC  Amplitude=0  Phase=0  Frequency=0  Measurements=None
  Controlled Voltage Source1 : powerlib/Electrical Sources/Controlled Voltage Source  Initialize=on  Source_Type=AC  Amplitude=0  Phase=0  Frequency=0  Measurements=None
  Controlled Voltage Source2 : powerlib/Electrical Sources/Controlled Voltage Source  Initialize=on  Source_Type=AC  Amplitude=0  Phase=0  Frequency=0  Measurements=None
  Current Measurement : powerlib/Measurements/Current Measurement  PhasorSimulation=off  OutputType=Complex  PSBequivalent=0
  Current Measurement1 : powerlib/Measurements/Current Measurement  PhasorSimulation=off  OutputType=Complex  PSBequivalent=0
  Current Measurement2 : powerlib/Measurements/Current Measurement  PhasorSimulation=off  OutputType=Complex  PSBequivalent=0
  Demux : Demux  Outputs=3
  Demux1 : Demux  Outputs=2
  Demux2 : Demux  Outputs=2
  Demux3 : Demux  Outputs=2
  Discrete-Time Integrator : DiscreteIntegrator  SampleTime=-1  ICPrevOutput=DiscIntNeverNeededParam  ICPrevScaledInput=DiscIntNeverNeededParam
  Discrete-Time Integrator1 : DiscreteIntegrator  SampleTime=-1  ICPrevOutput=DiscIntNeverNeededParam  ICPrevScaledInput=DiscIntNeverNeededParam
  Gain : Gain  Gain=psi_f
  Gain1 : Gain  Gain=psi_f
  Gain10 : Gain  Gain=Wbase
  Gain11 : Gain  Gain=1/Vbase
  Gain2 : Gain  Gain=L
  Gain3 : Gain  Gain=D
  Gain4 : Gain  Gain=1/J
  Gain5 : Gain  Gain=-psi_f
  Gain6 : Gain  Gain=psi_f
  Gain7 : Gain  Gain=Vbase
  Gain8 : Gain  Gain=1/(Sbase/Vbase)
  Integrator : Integrator
  Integrator1 : Integrator
  Manual Switch1 : ManualSwitch  CurrentSetting=0
  Manual Switch2 : ManualSwitch  CurrentSetting=0
  Manual Switch3 : ManualSwitch  CurrentSetting=0
  Math Function1 : Math  Operator=mod  SignedPower=on  SaturateOnIntegerOverflow=on
  Mux1 : Mux  Inputs=3
  Mux2 : Mux  Inputs=2
  Mux3 : Mux  Inputs=2
  Mux4 : Mux  Inputs=3
  Product{,1..3} (4 alike) : Product
  Trigonometric Function : Trigonometry
  Trigonometric Function1 : Trigonometry  Operator=cos
  Trigonometric Function2 : Trigonometry
  Trigonometric Function3 : Trigonometry  Operator=cos
  Voltage Measurement : powerlib/Measurements/Voltage Measurement  PhasorSimulation=off  OutputType=Complex  PSBequivalent=0
  Voltage Measurement1 : powerlib/Measurements/Voltage Measurement  PhasorSimulation=off  OutputType=Complex  PSBequivalent=0
  Voltage Measurement2 : powerlib/Measurements/Voltage Measurement  PhasorSimulation=off  OutputType=Complex  PSBequivalent=0
  Winding A : powerlib/Elements/Series RLC Branch  LConnTagsString=__new0  RConnTagsString=__new0  BranchType=RL  Resistance=R*(Vbase^2)/Sbase  Inductance=L*(Vbase^2)/Sbase/Wbase  SetiL0=off  InitialCurrent=ia0  Capacitance=1e-6  Setx0=off  InitialVoltage=0  Measurements=None
  Winding B : powerlib/Elements/Series RLC Branch  LConnTagsString=__new0  RConnTagsString=__new0  BranchType=RL  Resistance=R*(Vbase^2)/Sbase  Inductance=L*(Vbase^2)/Sbase/Wbase  SetiL0=off  InitialCurrent=ia0  Capacitance=1e-6  Setx0=off  InitialVoltage=0  Measurements=None
  Winding C : powerlib/Elements/Series RLC Branch  LConnTagsString=__new0  RConnTagsString=__new0  BranchType=RL  Resistance=R*(Vbase^2)/Sbase  Inductance=L*(Vbase^2)/Sbase/Wbase  SetiL0=off  InitialCurrent=ia0  Capacitance=1e-6  Setx0=off  InitialVoltage=0  Measurements=None
  "abc -> dq (Power-Invariant)1" : Subsystem  AncestorBlock=|
      | SimplusGT/Synchronous Machine
      | (dq-Frame System Object)/abc -> dq
      | (Power-Invariant)
  "abc -> dq (Power-Invariant)2" : Subsystem  AncestorBlock=|
      | SimplusGT/Synchronous Machine
      | (dq-Frame)
      | (Simulink Block)/abc -> dq
      | (Power-Invariant)1
  "dq -> abc (Power-Invariant)" : Subsystem  AncestorBlock=|
      | SimplusGT/dq -> abc
      | (Power-Invariant)
  a : PMIOPort  Side=Left
  b : PMIOPort  Port=2  Side=Left
  c : PMIOPort  Port=3  Side=Left
  n : PMIOPort  Port=4  Side=Left
  m : Outport
  wires:
  Current Measurement/1 -> Mux1/1
  Current Measurement1/1 -> Mux1/2
  Current Measurement2/1 -> Mux1/3
  Mux1/1 -> Gain8/1
  [e_abc] -> Gain7/1
  Demux/1 -> Controlled Voltage Source/1
  Demux/2 -> Controlled Voltage Source1/1
  Demux/3 -> Controlled Voltage Source2/1
  [i_abc] -> "abc -> dq (Power-Invariant)2"/1(abc)
  "abc -> dq (Power-Invariant)2"/1(dq) -> [i_dq]
  [w] -> Gain10/1
  Constant2/1 -> Add/2
  Trigonometric Function1/1 -> Gain1/1
  Trigonometric Function/1 -> Gain/1
  [i_dq] -> Gain2/1
  Demux1/1 -> Add1/2
  Demux1/2 -> Add2/1
  Gain2/1 -> Demux1/1
  Gain1/1 -> Add1/1
  Gain/1 -> Add2/2
  Product2/1 -> Mux2/1
  Product3/1 -> Mux2/2
  Mux2/1 -> [e_dq]
  [e_dq] -> "dq -> abc (Power-Invariant)"/1(dq)
  Add1/1 -> Mux3/1
  Add2/1 -> Mux3/2
  Mux3/1 -> [psi_dq]
  [psi_dq] -> Demux2/1
  [i_dq] -> Demux3/1
  Demux2/1 -> Product/1
  Demux3/2 -> Product/2
  Demux3/1 -> Product1/2
  Demux2/2 -> Product1/1
  Product/1 -> Add3/1
  Product1/1 -> Add3/2
  Add3/1 -> [Te]
  [Te] -> Add4/1
  Constant1/1 -> Add4/2
  Add4/1 -> Gain4/1
  Gain3/1 -> Add4/3
  Constant3/1 -> Add5/2
  Add5/1 -> Gain3/1, [w]
  Constant6/1 -> Trigonometric Function3/1, Trigonometric Function2/1
  Trigonometric Function2/1 -> Gain5/1
  Trigonometric Function3/1 -> Gain6/1
  Gain5/1 -> Product2/1
  Gain6/1 -> Product3/2
  Gain8/1 -> [i_abc]
  Gain4/1 -> Integrator1/1, Discrete-Time Integrator1/1
  Voltage Measurement/1 -> Mux4/1
  Voltage Measurement1/1 -> Mux4/2
  Voltage Measurement2/1 -> Mux4/3
  Mux4/1 -> Gain11/1
  Gain11/1 -> [v_abc]
  Gain7/1 -> Demux/1
  Add/1 -> Math Function1/1
  Constant4/1 -> Math Function1/2
  Math Function1/1 -> [theta]
  [v_abc] -> "abc -> dq (Power-Invariant)1"/1(abc)
  "abc -> dq (Power-Invariant)1"/1(dq) -> [v_dq]
  [w] -> Product3/1, Product2/2
  Constant5/1 -> Trigonometric Function/1, Trigonometric Function1/1
  Manual Switch1/1 -> Add5/1
  Constant10/1 -> Manual Switch1/1
  [theta] -> "dq -> abc (Power-Invariant)"/2(theta)
  [theta] -> "abc -> dq (Power-Invariant)2"/2(theta)
  [theta] -> "abc -> dq (Power-Invariant)1"/2(theta)
  [theta] -> Bus Creator/9  "theta"
  [e_dq] -> Bus Creator/4  "e_dq"
  [Te] -> Bus Creator/7  "Te"
  [i_abc] -> Bus Creator/3  "i_abc"
  [v_abc] -> Bus Creator/2  "v_abc"
  [v_dq] -> Bus Creator/5  "v_dq"
  [i_dq] -> Bus Creator/6  "i_dq"
  [e_abc] -> Bus Creator/1  "e_abc"
  [w] -> Bus Creator/8  "w"
  "dq -> abc (Power-Invariant)"/1(abc) -> [e_abc]
  Bus Creator/1 -> m/1
  Gain10/1 -> Discrete-Time Integrator/1, Integrator/1
  Integrator/1 -> Manual Switch2/2
  Manual Switch2/1 -> Add/1
  Discrete-Time Integrator/1 -> Manual Switch2/1
  Manual Switch3/1 -> Manual Switch1/2
  Integrator1/1 -> Manual Switch3/2
  Discrete-Time Integrator1/1 -> Manual Switch3/1
  connections:
  Current Measurement/RConn1 -- Winding A/RConn1
  Controlled Voltage Source/RConn1 -- Winding A/LConn1
  Current Measurement2/RConn1 -- Winding C/RConn1
  Current Measurement/LConn1 -- Voltage Measurement/LConn1 -- a/RConn1
  Current Measurement1/LConn1 -- Voltage Measurement1/LConn1 -- b/RConn1
  Current Measurement1/RConn1 -- Winding B/RConn1
  Winding B/LConn1 -- Controlled Voltage Source1/RConn1
  Controlled Voltage Source/LConn1 -- Voltage Measurement2/LConn2 -- Voltage Measurement1/LConn2 -- Voltage Measurement/LConn2 -- Controlled Voltage Source2/LConn1 -- n/RConn1 -- Controlled Voltage Source1/LConn1
  Winding C/LConn1 -- Controlled Voltage Source2/RConn1
  Current Measurement2/LConn1 -- Voltage Measurement2/LConn1 -- c/RConn1

== system SimplusGT_2020a/Three-Phase Bus ==
  note: Electrical Circuit
  note: Model for a three-phase bus.
      |
      | Author(s): Yitong Li
      |
      | Notes:
      |
      | It is simply a short-cuirt with current measurement. It is used in the toolbox model for highlighting the position of a bus and making the layout clearer.
  Mux : Mux  Inputs=3
  ia : powerlib/Measurements/Current Measurement  PhasorSimulation=off  OutputType=Complex  PSBequivalent=0
  ib : powerlib/Measurements/Current Measurement  PhasorSimulation=off  OutputType=Complex  PSBequivalent=0
  ic : powerlib/Measurements/Current Measurement  PhasorSimulation=off  OutputType=Complex  PSBequivalent=0
  a+ : PMIOPort  Side=Left
  -a : PMIOPort  Port=2  Side=Right
  b+ : PMIOPort  Port=3  Side=Left
  -b : PMIOPort  Port=4  Side=Right
  c+ : PMIOPort  Port=5  Side=Left
  -c : PMIOPort  Port=6  Side=Right
  wires:
  Mux/1 -> [iabc]
  ia/1 -> Mux/1
  ib/1 -> Mux/2
  ic/1 -> Mux/3
  connections:
  ic/RConn1 -- -c/RConn1
  ib/LConn1 -- b+/RConn1
  ib/RConn1 -- -b/RConn1
  ic/LConn1 -- c+/RConn1
  ia/LConn1 -- a+/RConn1
  ia/RConn1 -- -a/RConn1

== system SimplusGT_2020a/Three-Phase Signal ==
  note: Three-phase signal generator
      |
      | Author(s): Yitong Li
  Constant : Constant  Value=[ud uq]
  Constant1 : Constant  Value=w
  Constant2 : Constant  Value=theta0
  Constant3 : Constant  Value=2*pi
  Discrete-Time Integrator : DiscreteIntegrator  InitialConditionSource=external  SampleTime=Ts  ICPrevOutput=DiscIntNeverNeededParam  ICPrevScaledInput=DiscIntNeverNeededParam
  Math Function1 : Math  Operator=mod  SignedPower=on  SaturateOnIntegerOverflow=on
  "dq -> abc (Power-Invariant)" : Subsystem
  abc : Outport
  dq : Outport  Port=2
  theta : Outport  Port=3
  wires:
  Discrete-Time Integrator/1 -> Math Function1/1
  "dq -> abc (Power-Invariant)"/1(abc) -> abc/1
  Constant/1 -> "dq -> abc (Power-Invariant)"/1(dq), dq/1
  Math Function1/1 -> "dq -> abc (Power-Invariant)"/2(theta), theta/1
  Constant3/1 -> Math Function1/2
  Constant2/1 -> Discrete-Time Integrator/2
  Constant1/1 -> Discrete-Time Integrator/1

== system SimplusGT_2020a/Three-Phase Signal (Advanced) ==
  note: Three-phase signal generator
      |
      | Author(s): Yitong Li
      |
      | Notes:
      |
      | This block has advanced settings.
  Constant : Constant  Value=[ud uq]
  Constant1 : Constant  Value=w
  Constant2 : Constant  Value=theta0
  Constant3 : Constant  Value=2*pi
  Constant4 : Constant  Value=enable_freq_step
  Discrete-Time Integrator : DiscreteIntegrator  InitialConditionSource=external  SampleTime=Ts  ICPrevOutput=DiscIntNeverNeededParam  ICPrevScaledInput=DiscIntNeverNeededParam
  Math Function1 : Math  Operator=mod  SignedPower=on  SaturateOnIntegerOverflow=on
  Product : Product
  Step : Step  Time=time_freq_step  Before=1  After=ratio_freq_step  SampleTime=0
  Switch : Switch  Criteria=u2 > Threshold  Threshold=0.5
  "dq -> abc (Power-Invariant)1" : SimplexPS_2015a/Three-Phase Signal/dq -> abc (Power-Invariant)  SystemSampleTime=-1  Latency=0  AutoFrameSizeCalculation=off
  abc : Outport
  dq : Outport  Port=2
  theta : Outport  Port=3
  wires:
  Constant3/1 -> Math Function1/2
  Constant4/1 -> Switch/2
  Switch/1 -> Discrete-Time Integrator/1
  Constant1/1 -> Product/2, Switch/3
  Constant2/1 -> Discrete-Time Integrator/2
  Product/1 -> Switch/1
  Math Function1/1 -> theta/1, "dq -> abc (Power-Invariant)1"/2
  Constant/1 -> dq/1, "dq -> abc (Power-Invariant)1"/1
  Discrete-Time Integrator/1 -> Math Function1/1
  "dq -> abc (Power-Invariant)1"/1 -> abc/1
  Step/1 -> Product/1

== system SimplusGT_2020a/Timer ==
  note: Timer
      |
      | Author(s): Yitong Li
  Constant : Constant
  Discrete-Time Integrator : DiscreteIntegrator  SampleTime=Ts  ICPrevOutput=DiscIntNeverNeededParam  ICPrevScaledInput=DiscIntNeverNeededParam
  Gain : Gain
  Gain1 : Gain  Gain=1/60
  Gain2 : Gain  Gain=1/60
  sec : Outport
  min : Outport  Port=2
  h : Outport  Port=3
  wires:
  Constant/1 -> Discrete-Time Integrator/1
  Discrete-Time Integrator/1 -> Gain/1
  Gain/1 -> Gain1/1, sec/1
  Gain1/1 -> Gain2/1, min/1
  Gain2/1 -> h/1

== system SimplusGT_2020a/Two-Phase Bus ==
  note: Electrical Circuit
  note: Model for a two-phase bus.
      |
      | Author(s): Yitong Li
      |
      | Notes:
      |
      | It is simply a short-cuirt with current measurement. It is used in the toolbox model for highlighting the position of a bus and making the layout clearer.
  Mux : Mux  Inputs=2
  ia : powerlib/Measurements/Current Measurement  PhasorSimulation=off  OutputType=Complex  PSBequivalent=0
  ib : powerlib/Measurements/Current Measurement  PhasorSimulation=off  OutputType=Complex  PSBequivalent=0
  a+ : PMIOPort  Side=Left
  -a : PMIOPort  Port=2  Side=Right
  b+ : PMIOPort  Port=3  Side=Left
  -b : PMIOPort  Port=4  Side=Right
  wires:
  Mux/1 -> [iab]
  ia/1 -> Mux/1
  ib/1 -> Mux/2
  connections:
  ib/LConn1 -- b+/RConn1
  ib/RConn1 -- -b/RConn1
  ia/LConn1 -- a+/RConn1
  ia/RConn1 -- -a/RConn1

== system SimplusGT_2020a/Voltage Measurement (2ph -> 3ph) ==
  note: Three-phase voltage measurement.
      |
      | Author(s): Yitong Li
      |
      | Notes:
      |
      | vc is calculated from va and vb with assuming that va + vb + vc = 0.
  Add : Sum  Inputs=--+
  Constant : Constant  Value=0
  Mux : Mux  Inputs=3
  va : powerlib/Measurements/Voltage Measurement  PhasorSimulation=off  OutputType=Complex  PSBequivalent=0
  vb : powerlib/Measurements/Voltage Measurement  PhasorSimulation=off  OutputType=Complex  PSBequivalent=0
  a : PMIOPort  Side=Left
  b : PMIOPort  Port=2  Side=Left
  n : PMIOPort  Port=3  Side=Left
  vabc : Outport
  wires:
  Mux/1 -> vabc/1
  va/1 -> Mux/1, Add/1
  vb/1 -> Mux/2, Add/2
  Constant/1 -> Add/3
  Add/1 -> Mux/3
  connections:
  vb/LConn2 -- va/LConn2 -- n/RConn1
  vb/LConn1 -- b/RConn1
  va/LConn1 -- a/RConn1

== system SimplusGT_2020a/Voltage Measurement (3ph -> 3ph) ==
  note: Three-phase voltage measurement.
      |
      | Author(s): Yitong Li
  Mux : Mux  Inputs=3
  va : powerlib/Measurements/Voltage Measurement  PhasorSimulation=off  OutputType=Complex  PSBequivalent=0
  vb : powerlib/Measurements/Voltage Measurement  PhasorSimulation=off  OutputType=Complex  PSBequivalent=0
  vc : powerlib/Measurements/Voltage Measurement  PhasorSimulation=off  OutputType=Complex  PSBequivalent=0
  a : PMIOPort  Side=Left
  b : PMIOPort  Port=2  Side=Left
  c : PMIOPort  Port=3  Side=Left
  n : PMIOPort  Port=4  Side=Left
  vabc : Outport
  wires:
  vc/1 -> Mux/3
  Mux/1 -> vabc/1
  va/1 -> Mux/1
  vb/1 -> Mux/2
  connections:
  vb/LConn2 -- va/LConn2 -- vc/LConn2 -- n/RConn1
  vc/LConn1 -- c/RConn1
  vb/LConn1 -- b/RConn1
  va/LConn1 -- a/RConn1

== system SimplusGT_2020a/Voltage Disturbance ==
  note: Model for a voltage disturbance.
      |
      | Author(s): Yitong Li
  vabc : Inport
  Controlled Voltage Source : powerlib/Electrical Sources/Controlled Voltage Source  Initialize=on  Source_Type=AC  Amplitude=0  Phase=0  Frequency=0  Measurements=None
  Controlled Voltage Source1 : powerlib/Electrical Sources/Controlled Voltage Source  Initialize=on  Source_Type=AC  Amplitude=0  Phase=0  Frequency=0  Measurements=None
  Controlled Voltage Source2 : powerlib/Electrical Sources/Controlled Voltage Source  Initialize=on  Source_Type=AC  Amplitude=0  Phase=0  Frequency=0  Measurements=None
  Demux : Demux  Outputs=3
  Gain : Gain  Gain=Vbase
  a+ : PMIOPort  Side=Right
  a- : PMIOPort  Port=2  Side=Left
  b+ : PMIOPort  Port=3  Side=Right
  b- : PMIOPort  Port=4  Side=Left
  c+ : PMIOPort  Port=5  Side=Right
  c- : PMIOPort  Port=6  Side=Left
  wires:
  vabc/1 -> Gain/1
  Demux/1 -> Controlled Voltage Source/1
  Demux/2 -> Controlled Voltage Source1/1
  Demux/3 -> Controlled Voltage Source2/1
  Gain/1 -> Demux/1
  connections:
  Controlled Voltage Source2/LConn1 -- c-/RConn1
  Controlled Voltage Source1/RConn1 -- b+/RConn1
  Controlled Voltage Source2/RConn1 -- c+/RConn1
  Controlled Voltage Source/RConn1 -- a+/RConn1
  Controlled Voltage Source/LConn1 -- a-/RConn1
  Controlled Voltage Source1/LConn1 -- b-/RConn1
